simulink model "Pr2"  (R2022b)
settings: Solver=VariableStepAuto  StartTime=0.0  StopTime=30.0  RelTol=1e-3
settings Model: Creator=rus_d  LastModifiedBy=rus_d

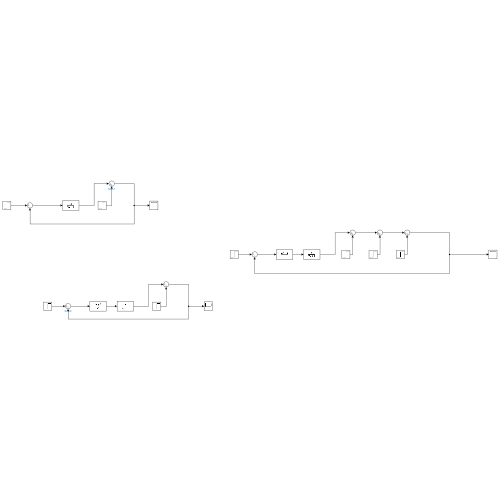
[thumbnail: Simulink's stored preview of the top-level diagram]
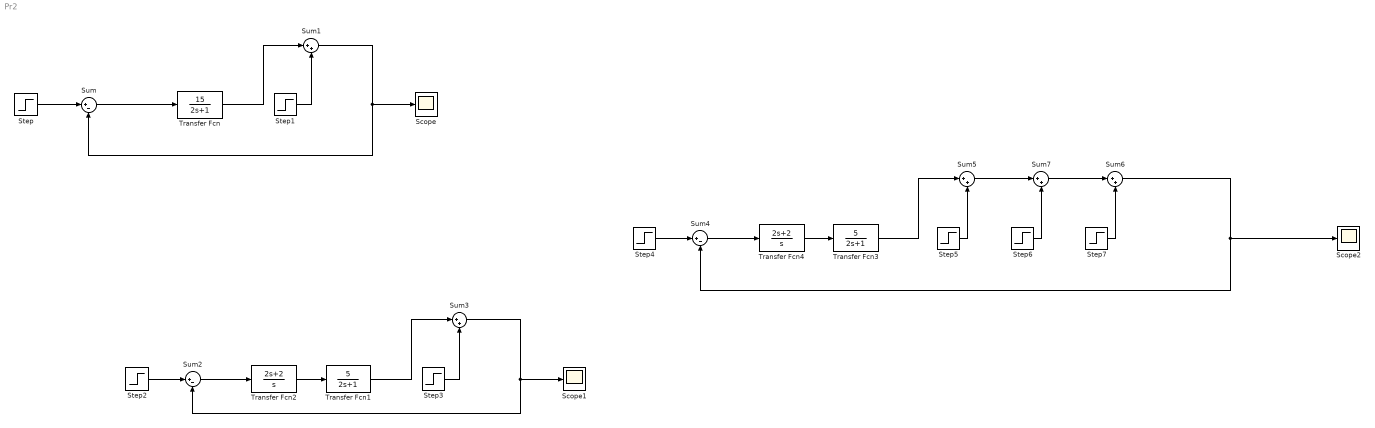
== system Pr2 ==
  Scope : Scope
  Scope1 : Scope
  Scope2 : Scope
  Step : Step  SampleTime=0
  Step1 : Step  Time=5  After=0.5  SampleTime=0
  Step2 : Step  SampleTime=0
  Step3 : Step  Time=5  After=0.5  SampleTime=0
  Step4 : Step  SampleTime=0
  Step5 : Step  Time=5  After=0.2  SampleTime=0
  Step6 : Step  Time=10  After=0.3  SampleTime=0
  Step7 : Step  Time=15  After=0.4  SampleTime=0
  Sum : Sum  Inputs=|+-
  Sum{1,3,5..7} (5 alike) : Sum  Inputs=|++
  Sum2 : Sum  Inputs=|+-
  Sum4 : Sum  Inputs=|+-
  Transfer Fcn : TransferFcn  Numerator=[15]  Denominator=[2 1]
  Transfer Fcn1 : TransferFcn  Numerator=[5]  Denominator=[2 1]
  Transfer Fcn2 : TransferFcn  Numerator=[2 2]  Denominator=[1 0]
  Transfer Fcn3 : TransferFcn  Numerator=[5]  Denominator=[2 1]
  Transfer Fcn4 : TransferFcn  Numerator=[2 2]  Denominator=[1 0]
  wires:
  Step/1 -> Sum/1
  Sum/1 -> Transfer Fcn/1
  Transfer Fcn/1 -> Sum1/1
  Sum1/1 -> Sum/2, Scope/1
  Step1/1 -> Sum1/2
  Step3/1 -> Sum3/2
  Sum3/1 -> Sum2/2, Scope1/1
  Step2/1 -> Sum2/1
  Transfer Fcn1/1 -> Sum3/1
  Sum2/1 -> Transfer Fcn2/1
  Transfer Fcn2/1 -> Transfer Fcn1/1
  Sum4/1 -> Transfer Fcn4/1
  Step5/1 -> Sum5/2
  Step4/1 -> Sum4/1
  Transfer Fcn3/1 -> Sum5/1
  Transfer Fcn4/1 -> Transfer Fcn3/1
  Sum5/1 -> Sum7/1
  Sum7/1 -> Sum6/1
  Sum6/1 -> Scope2/1, Sum4/2
  Step6/1 -> Sum7/2
  Step7/1 -> Sum6/2
